simulink model "IFFT64K_2D"  (R2023a)
settings: Solver=VariableStepAuto  StartTime=0.0  StopTime=simtime  RelTol=1e-3
PostLoadFcn:
  | samp_rate = 2e9;
  | fft_sz = 65536;
  | chirp_rate = 200e6 / 1e-3;
  | tone_freq = 20e6;
  | input_bits = 12;
  | align_delay = 3 * fft_sz;
  | buff_init = complex(int32(zeros(256,1)));
  | NSTREAM = 5;
  | simtime = 2.5e-4;
undefined symbols (not defined in the file): S, vsva2197, xcvc1902
libraries: aieBasic x30, aieUtilities x15, hlsBasic x1, dspxfrm3 x1, dspsrcs4 x1, vmcUtilities x1
(part 2 of 2)

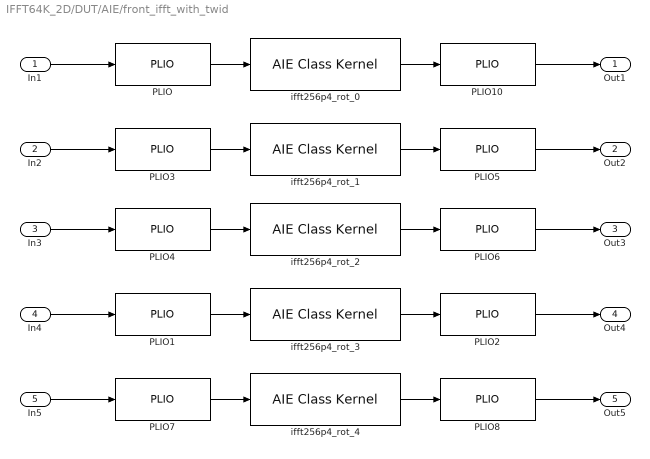
== system IFFT64K_2D/DUT/AIE/front_ifft_with_twid ==
  In1 : Inport
  In2 : Inport  Port=2
  In3 : Inport  Port=3
  In4 : Inport  Port=4
  In5 : Inport  Port=5
  PLIO{,1..8,10} (10 alike) : aieBasic/PLIO  PlioWidth=64  PlioFreqSpec=off  PlioFreq=250  ColLocation=0  channel=0  blockJsonConstraints=[]  deprecateConstraints=0
  ifft256p4_rot_0 : aieBasic/AIE Class Kernel  KernelAllAttrs=|  PortNames={'sig_i'; 'sig_o'}  PortSerializedTypes={'{Q2{R{Tadf::input_buffer{2{t{Scint32}}{t{Tadf::extents{1{t{}260}}}}}}}}'; '{Q2{R{Tadf::output_buffer{2{t{Scint32}}{t{Tadf::extents{1{t{}260}}}}}}}}'}  PortWindowSizes={2.600000000000000000e+02; 2.600000000000000000e+02}  PortWindowMargins={0.000000000000000000e+00; 0.000000000000000000e+00}  PortSynchronicities={'sync', 'sync'}  PortSignalSizes={0.000000000000000000e+00; 0.000000000000000000e+00}  ClassTemplateSpecKind=implicit  ClassTemplateParamNames={'NSTREAM'; 'PHASE'}  ClassTemplateParamKinds={'nontype'; 'nontype'}  ClassTemplateParamTypes={'unsigned int'; 'unsigned int'}  ClassTemplateParamValues={'5', '4'}  ClassCtorParamNames={'tbuff_i'}  ClassCtorParamSerializedTypes={'{R{C{Scint32}256}}'}  ClassCtorParamValues={'[0;0;0;0;0;0;0;0;0;0;0;0;0;0;0;0;0;0;0;0;0;0;0;0;0;0;0;0;0;0;0;0;0;0;0;0;0;0;0;0;0;0;0;0;0;0;0;0;0;0;0;0;0;0;0;0;0;0;0;0;0;0;0;0;0;0;0;0;0;0;0;0;0;0;0;0;0;0;0;0;0;0;0;0;0;0;0;0;0;0;0;0;0;0;0;0;0;0;0;0;0;0;0;0;0;0;0;0;0;0;0;0;0;0;0;0;0;0;0;0;0;0;0;0;0;0;0;0;0;0;0;0;0;0;0;0;0;0;0;0;0;0;0;0;0;0;0;0;0;0;0;0;0;0;0;0;0;0;0;0;0;0;0;0;0;0;0;0;0;0;0;0;0;0;0;0;0;0;0;0;0;0;0;0;0;0;0;0;0;0;0;0;0;0;0;0;0;0;0;0;0;0;0;0;0;0;0;0;0;0;0;0;0;0;0;0;0;0;0;0;0;0;0;0;0;0;0;0;0;0;0;0;0;0;0;0;0;0;0;0;0;0;0;0;0;0;0;0;0;0;0;0;0;0;0;0]'}  ClassIndex=1  ClassCtorIndex=1  ClassTabVisible=on  ClassTemplateParamsVisible=on  ClassCtorDeclVisible=on  ClassCtorParamsVisible=on  FunctionTabVisible=on  FunctionDecl=|  PortAttrs={ 'input', 'sig_i', 'adf::input_buffer< cint32, adf::extents< 260 > > & restrict', '260', '0', 'sync', ''; 'output', 'sig_o', 'adf::output_buffer< cint32, adf::extents< 260 > > & restrict', '260', '', 'sync', '' }  PortAttrsEnables={'off', 'off', 'off', 'off', 'off', 'off', 'off';'off', 'off', 'off', 'off', 'off', 'off', 'off'}  SampleTime=-1  ClassDeclTypeOptions=C[1 1]@t74@template < unsigned int NSTREAM, unsigned int PHASE > class ifft256p4_rot;  ClassDecl=template < unsigned int NSTREAM, unsigned int PHASE > class ifft256p4_rot;  ClassTemplateParams={ 'NSTREAM', 'unsigned int', 'NSTREAM'; 'PHASE', 'unsigned int', '4' }  ClassTemplateParamsEnables={'off', 'off', 'on';'off', 'off', 'on'}  ClassCtorDeclTypeOptions=C[1 1]@t43@ifft256p4_rot(cint32 ( & tbuff_i ) [ 256 ])  ClassCtorDecl=ifft256p4_rot(cint32 ( & tbuff_i ) [ 256 ])  ClassCtorParams={ 'tbuff_i', 'cint32 ( &) [ 256 ]', 'buff_init' }  KernelHeaderFile=aie_src/ifft256p4_rot.h  KernelClassName=ifft256p4_rot  KernelFunction=run  KernelSourceFile=aie_src/ifft256p4_rot.cpp  KernelSearchPaths={}  PreProcOptions={}  blockJsonConstraints=[]
      KernelAllAttrs=|
      | s[12;12;9;9;19;14;21;23;21;23;24;21;15;17;12;24;26;26;26;27;28;9;21;23;23;23;24;25;14;19;19;29]@FunctionNameDeclFileNamePortNamesPortTypesPortSerializedTypesPortDirectionsPortWindowSizeEnablesPortWindowMarginEnablesPortBufferSizeEnablesPortBufferMarginEnablesPortSynchronicityEnablesPortSignalSizeEnablesPortBufferSizesPortBufferMarginsFunctionDeclFunctionTemplateSpecKindFunctionTemplateParamNamesFunctionTemplateParamKindsFunctionTemplateParamTypesFunctionTemplateParamValuesFunctionTemplateParamEnablesClassDeclClassTemplateSpecKindClassTemplateParamNamesClassTemplateParamKindsClassTemplateParamTypesClassTemplateParamValuesClassTemplateParamEnablesClassCtorDeclsClassCtorParamNamesClassCtorParamTypesClassCtorParamSerializedTypes[1 1]@C[32 1]@t3@runt33@../../aie_src/ifft256p4_rot_vmc.hC[2 1]@t5@sig_it5@sig_oC[2 1]@t59@adf::input_buffer< cint32, adf::extents< 260 > > & restrictt60@adf::output_buffer< cint32, adf::extents< 260 > > & restrictC[2 1]@t71@{Q2{R{Tadf::input_buffer{2{t{Scint32}}{t{Tadf::extents{1{t{}260}}}}}}}}t72@{Q2{R{Tadf::output_buffer{2{t{Scint32}}{t{Tadf::extents{1{t{}260}}}}}}}}C[2 1]@t5@inputt6@outputC[2 1]@l1@l1@C[2 1]@l1@l0@C[2 1]@l1@l1@C[2 1]@l0@l0@C[2 1]@l1@l1@C[2 1]@l0@l0@C[2 1]@t3@260t3@260C[2 1]@nnt214@template < unsigned int NSTREAM, unsigned int PHASE > 
      | void ifft256p4_rot::
      | run(adf::input_buffer< cint32, adf::extents< 260 > > & restrict sig_i, adf::output_buffer< cint32, adf::extents< 260 > > & restrict sig_o)t4@nonee[0 1]@e[0 1]@e[0 1]@e[0 1]@e[0 1]@t74@template < unsigned int NSTREAM, unsigned int PHASE > class ifft256p4_rot;t8@implicitC[2 1]@t7@NSTREAMt5@PHASEC[2 1]@t7@nontypet7@nontypeC[2 1]@t12@unsigned intt12@unsigned intC[2 1]@nnC[2 1]@l1@l1@C[1 1]@t43@ifft256p4_rot(cint32 ( & tbuff_i ) [ 256 ])C[1 1]@C[1 1]@t7@tbuff_iC[1 1]@C[1 1]@t19@cint32 ( &) [ 256 ]C[1 1]@C[1 1]@t18@{R{C{Scint32}256}}
      FunctionDecl=|
      | template < unsigned int NSTREAM, unsigned int PHASE > 
      | void ifft256p4_rot::
      | run(adf::input_buffer< cint32, adf::extents< 260 > > & restrict sig_i, adf::output_buffer< cint32, adf::extents< 260 > > & restrict sig_o)
  ifft256p4_rot_1 : aieBasic/AIE Class Kernel  KernelAllAttrs=|  PortNames={'sig_i'; 'sig_o'}  PortSerializedTypes={'{Q2{R{Tadf::input_buffer{2{t{Scint32}}{t{Tadf::extents{1{t{}260}}}}}}}}'; '{Q2{R{Tadf::output_buffer{2{t{Scint32}}{t{Tadf::extents{1{t{}260}}}}}}}}'}  PortWindowSizes={2.600000000000000000e+02; 2.600000000000000000e+02}  PortWindowMargins={0.000000000000000000e+00; 0.000000000000000000e+00}  PortSynchronicities={'sync', 'sync'}  PortSignalSizes={0.000000000000000000e+00; 0.000000000000000000e+00}  ClassTemplateSpecKind=implicit  ClassTemplateParamNames={'NSTREAM'; 'PHASE'}  ClassTemplateParamKinds={'nontype'; 'nontype'}  ClassTemplateParamTypes={'unsigned int'; 'unsigned int'}  ClassTemplateParamValues={'5', '4'}  ClassCtorParamNames={'tbuff_i'}  ClassCtorParamSerializedTypes={'{R{C{Scint32}256}}'}  ClassCtorParamValues={'[0;0;0;0;0;0;0;0;0;0;0;0;0;0;0;0;0;0;0;0;0;0;0;0;0;0;0;0;0;0;0;0;0;0;0;0;0;0;0;0;0;0;0;0;0;0;0;0;0;0;0;0;0;0;0;0;0;0;0;0;0;0;0;0;0;0;0;0;0;0;0;0;0;0;0;0;0;0;0;0;0;0;0;0;0;0;0;0;0;0;0;0;0;0;0;0;0;0;0;0;0;0;0;0;0;0;0;0;0;0;0;0;0;0;0;0;0;0;0;0;0;0;0;0;0;0;0;0;0;0;0;0;0;0;0;0;0;0;0;0;0;0;0;0;0;0;0;0;0;0;0;0;0;0;0;0;0;0;0;0;0;0;0;0;0;0;0;0;0;0;0;0;0;0;0;0;0;0;0;0;0;0;0;0;0;0;0;0;0;0;0;0;0;0;0;0;0;0;0;0;0;0;0;0;0;0;0;0;0;0;0;0;0;0;0;0;0;0;0;0;0;0;0;0;0;0;0;0;0;0;0;0;0;0;0;0;0;0;0;0;0;0;0;0;0;0;0;0;0;0;0;0;0;0;0;0]'}  ClassIndex=1  ClassCtorIndex=1  ClassTabVisible=on  ClassTemplateParamsVisible=on  ClassCtorDeclVisible=on  ClassCtorParamsVisible=on  FunctionTabVisible=on  FunctionDecl=|  PortAttrs={ 'input', 'sig_i', 'adf::input_buffer< cint32, adf::extents< 260 > > & restrict', '260', '0', 'sync', ''; 'output', 'sig_o', 'adf::output_buffer< cint32, adf::extents< 260 > > & restrict', '260', '', 'sync', '' }  PortAttrsEnables={'off', 'off', 'off', 'off', 'off', 'off', 'off';'off', 'off', 'off', 'off', 'off', 'off', 'off'}  SampleTime=-1  ClassDeclTypeOptions=C[1 1]@t74@template < unsigned int NSTREAM, unsigned int PHASE > class ifft256p4_rot;  ClassDecl=template < unsigned int NSTREAM, unsigned int PHASE > class ifft256p4_rot;  ClassTemplateParams={ 'NSTREAM', 'unsigned int', 'NSTREAM'; 'PHASE', 'unsigned int', '4' }  ClassTemplateParamsEnables={'off', 'off', 'on';'off', 'off', 'on'}  ClassCtorDeclTypeOptions=C[1 1]@t43@ifft256p4_rot(cint32 ( & tbuff_i ) [ 256 ])  ClassCtorDecl=ifft256p4_rot(cint32 ( & tbuff_i ) [ 256 ])  ClassCtorParams={ 'tbuff_i', 'cint32 ( &) [ 256 ]', 'buff_init' }  KernelHeaderFile=aie_src/ifft256p4_rot.h  KernelClassName=ifft256p4_rot  KernelFunction=run  KernelSourceFile=aie_src/ifft256p4_rot.cpp  KernelSearchPaths={}  PreProcOptions={}  blockJsonConstraints=[]
      KernelAllAttrs=|
      | s[12;12;9;9;19;14;21;23;21;23;24;21;15;17;12;24;26;26;26;27;28;9;21;23;23;23;24;25;14;19;19;29]@FunctionNameDeclFileNamePortNamesPortTypesPortSerializedTypesPortDirectionsPortWindowSizeEnablesPortWindowMarginEnablesPortBufferSizeEnablesPortBufferMarginEnablesPortSynchronicityEnablesPortSignalSizeEnablesPortBufferSizesPortBufferMarginsFunctionDeclFunctionTemplateSpecKindFunctionTemplateParamNamesFunctionTemplateParamKindsFunctionTemplateParamTypesFunctionTemplateParamValuesFunctionTemplateParamEnablesClassDeclClassTemplateSpecKindClassTemplateParamNamesClassTemplateParamKindsClassTemplateParamTypesClassTemplateParamValuesClassTemplateParamEnablesClassCtorDeclsClassCtorParamNamesClassCtorParamTypesClassCtorParamSerializedTypes[1 1]@C[32 1]@t3@runt33@../../aie_src/ifft256p4_rot_vmc.hC[2 1]@t5@sig_it5@sig_oC[2 1]@t59@adf::input_buffer< cint32, adf::extents< 260 > > & restrictt60@adf::output_buffer< cint32, adf::extents< 260 > > & restrictC[2 1]@t71@{Q2{R{Tadf::input_buffer{2{t{Scint32}}{t{Tadf::extents{1{t{}260}}}}}}}}t72@{Q2{R{Tadf::output_buffer{2{t{Scint32}}{t{Tadf::extents{1{t{}260}}}}}}}}C[2 1]@t5@inputt6@outputC[2 1]@l1@l1@C[2 1]@l1@l0@C[2 1]@l1@l1@C[2 1]@l0@l0@C[2 1]@l1@l1@C[2 1]@l0@l0@C[2 1]@t3@260t3@260C[2 1]@nnt214@template < unsigned int NSTREAM, unsigned int PHASE > 
      | void ifft256p4_rot::
      | run(adf::input_buffer< cint32, adf::extents< 260 > > & restrict sig_i, adf::output_buffer< cint32, adf::extents< 260 > > & restrict sig_o)t4@nonee[0 1]@e[0 1]@e[0 1]@e[0 1]@e[0 1]@t74@template < unsigned int NSTREAM, unsigned int PHASE > class ifft256p4_rot;t8@implicitC[2 1]@t7@NSTREAMt5@PHASEC[2 1]@t7@nontypet7@nontypeC[2 1]@t12@unsigned intt12@unsigned intC[2 1]@nnC[2 1]@l1@l1@C[1 1]@t43@ifft256p4_rot(cint32 ( & tbuff_i ) [ 256 ])C[1 1]@C[1 1]@t7@tbuff_iC[1 1]@C[1 1]@t19@cint32 ( &) [ 256 ]C[1 1]@C[1 1]@t18@{R{C{Scint32}256}}
      FunctionDecl=|
      | template < unsigned int NSTREAM, unsigned int PHASE > 
      | void ifft256p4_rot::
      | run(adf::input_buffer< cint32, adf::extents< 260 > > & restrict sig_i, adf::output_buffer< cint32, adf::extents< 260 > > & restrict sig_o)
  ifft256p4_rot_2 : aieBasic/AIE Class Kernel  KernelAllAttrs=|  PortNames={'sig_i'; 'sig_o'}  PortSerializedTypes={'{Q2{R{Tadf::input_buffer{2{t{Scint32}}{t{Tadf::extents{1{t{}260}}}}}}}}'; '{Q2{R{Tadf::output_buffer{2{t{Scint32}}{t{Tadf::extents{1{t{}260}}}}}}}}'}  PortWindowSizes={2.600000000000000000e+02; 2.600000000000000000e+02}  PortWindowMargins={0.000000000000000000e+00; 0.000000000000000000e+00}  PortSynchronicities={'sync', 'sync'}  PortSignalSizes={0.000000000000000000e+00; 0.000000000000000000e+00}  ClassTemplateSpecKind=implicit  ClassTemplateParamNames={'NSTREAM'; 'PHASE'}  ClassTemplateParamKinds={'nontype'; 'nontype'}  ClassTemplateParamTypes={'unsigned int'; 'unsigned int'}  ClassTemplateParamValues={'5', '4'}  ClassCtorParamNames={'tbuff_i'}  ClassCtorParamSerializedTypes={'{R{C{Scint32}256}}'}  ClassCtorParamValues={'[0;0;0;0;0;0;0;0;0;0;0;0;0;0;0;0;0;0;0;0;0;0;0;0;0;0;0;0;0;0;0;0;0;0;0;0;0;0;0;0;0;0;0;0;0;0;0;0;0;0;0;0;0;0;0;0;0;0;0;0;0;0;0;0;0;0;0;0;0;0;0;0;0;0;0;0;0;0;0;0;0;0;0;0;0;0;0;0;0;0;0;0;0;0;0;0;0;0;0;0;0;0;0;0;0;0;0;0;0;0;0;0;0;0;0;0;0;0;0;0;0;0;0;0;0;0;0;0;0;0;0;0;0;0;0;0;0;0;0;0;0;0;0;0;0;0;0;0;0;0;0;0;0;0;0;0;0;0;0;0;0;0;0;0;0;0;0;0;0;0;0;0;0;0;0;0;0;0;0;0;0;0;0;0;0;0;0;0;0;0;0;0;0;0;0;0;0;0;0;0;0;0;0;0;0;0;0;0;0;0;0;0;0;0;0;0;0;0;0;0;0;0;0;0;0;0;0;0;0;0;0;0;0;0;0;0;0;0;0;0;0;0;0;0;0;0;0;0;0;0;0;0;0;0;0;0]'}  ClassIndex=1  ClassCtorIndex=1  ClassTabVisible=on  ClassTemplateParamsVisible=on  ClassCtorDeclVisible=on  ClassCtorParamsVisible=on  FunctionTabVisible=on  FunctionDecl=|  PortAttrs={ 'input', 'sig_i', 'adf::input_buffer< cint32, adf::extents< 260 > > & restrict', '260', '0', 'sync', ''; 'output', 'sig_o', 'adf::output_buffer< cint32, adf::extents< 260 > > & restrict', '260', '', 'sync', '' }  PortAttrsEnables={'off', 'off', 'off', 'off', 'off', 'off', 'off';'off', 'off', 'off', 'off', 'off', 'off', 'off'}  SampleTime=-1  ClassDeclTypeOptions=C[1 1]@t74@template < unsigned int NSTREAM, unsigned int PHASE > class ifft256p4_rot;  ClassDecl=template < unsigned int NSTREAM, unsigned int PHASE > class ifft256p4_rot;  ClassTemplateParams={ 'NSTREAM', 'unsigned int', 'NSTREAM'; 'PHASE', 'unsigned int', '4' }  ClassTemplateParamsEnables={'off', 'off', 'on';'off', 'off', 'on'}  ClassCtorDeclTypeOptions=C[1 1]@t43@ifft256p4_rot(cint32 ( & tbuff_i ) [ 256 ])  ClassCtorDecl=ifft256p4_rot(cint32 ( & tbuff_i ) [ 256 ])  ClassCtorParams={ 'tbuff_i', 'cint32 ( &) [ 256 ]', 'buff_init' }  KernelHeaderFile=aie_src/ifft256p4_rot.h  KernelClassName=ifft256p4_rot  KernelFunction=run  KernelSourceFile=aie_src/ifft256p4_rot.cpp  KernelSearchPaths={}  PreProcOptions={}  blockJsonConstraints=[]
      KernelAllAttrs=|
      | s[12;12;9;9;19;14;21;23;21;23;24;21;15;17;12;24;26;26;26;27;28;9;21;23;23;23;24;25;14;19;19;29]@FunctionNameDeclFileNamePortNamesPortTypesPortSerializedTypesPortDirectionsPortWindowSizeEnablesPortWindowMarginEnablesPortBufferSizeEnablesPortBufferMarginEnablesPortSynchronicityEnablesPortSignalSizeEnablesPortBufferSizesPortBufferMarginsFunctionDeclFunctionTemplateSpecKindFunctionTemplateParamNamesFunctionTemplateParamKindsFunctionTemplateParamTypesFunctionTemplateParamValuesFunctionTemplateParamEnablesClassDeclClassTemplateSpecKindClassTemplateParamNamesClassTemplateParamKindsClassTemplateParamTypesClassTemplateParamValuesClassTemplateParamEnablesClassCtorDeclsClassCtorParamNamesClassCtorParamTypesClassCtorParamSerializedTypes[1 1]@C[32 1]@t3@runt33@../../aie_src/ifft256p4_rot_vmc.hC[2 1]@t5@sig_it5@sig_oC[2 1]@t59@adf::input_buffer< cint32, adf::extents< 260 > > & restrictt60@adf::output_buffer< cint32, adf::extents< 260 > > & restrictC[2 1]@t71@{Q2{R{Tadf::input_buffer{2{t{Scint32}}{t{Tadf::extents{1{t{}260}}}}}}}}t72@{Q2{R{Tadf::output_buffer{2{t{Scint32}}{t{Tadf::extents{1{t{}260}}}}}}}}C[2 1]@t5@inputt6@outputC[2 1]@l1@l1@C[2 1]@l1@l0@C[2 1]@l1@l1@C[2 1]@l0@l0@C[2 1]@l1@l1@C[2 1]@l0@l0@C[2 1]@t3@260t3@260C[2 1]@nnt214@template < unsigned int NSTREAM, unsigned int PHASE > 
      | void ifft256p4_rot::
      | run(adf::input_buffer< cint32, adf::extents< 260 > > & restrict sig_i, adf::output_buffer< cint32, adf::extents< 260 > > & restrict sig_o)t4@nonee[0 1]@e[0 1]@e[0 1]@e[0 1]@e[0 1]@t74@template < unsigned int NSTREAM, unsigned int PHASE > class ifft256p4_rot;t8@implicitC[2 1]@t7@NSTREAMt5@PHASEC[2 1]@t7@nontypet7@nontypeC[2 1]@t12@unsigned intt12@unsigned intC[2 1]@nnC[2 1]@l1@l1@C[1 1]@t43@ifft256p4_rot(cint32 ( & tbuff_i ) [ 256 ])C[1 1]@C[1 1]@t7@tbuff_iC[1 1]@C[1 1]@t19@cint32 ( &) [ 256 ]C[1 1]@C[1 1]@t18@{R{C{Scint32}256}}
      FunctionDecl=|
      | template < unsigned int NSTREAM, unsigned int PHASE > 
      | void ifft256p4_rot::
      | run(adf::input_buffer< cint32, adf::extents< 260 > > & restrict sig_i, adf::output_buffer< cint32, adf::extents< 260 > > & restrict sig_o)
  ifft256p4_rot_3 : aieBasic/AIE Class Kernel  KernelAllAttrs=|  PortNames={'sig_i'; 'sig_o'}  PortSerializedTypes={'{Q2{R{Tadf::input_buffer{2{t{Scint32}}{t{Tadf::extents{1{t{}260}}}}}}}}'; '{Q2{R{Tadf::output_buffer{2{t{Scint32}}{t{Tadf::extents{1{t{}260}}}}}}}}'}  PortWindowSizes={2.600000000000000000e+02; 2.600000000000000000e+02}  PortWindowMargins={0.000000000000000000e+00; 0.000000000000000000e+00}  PortSynchronicities={'sync', 'sync'}  PortSignalSizes={0.000000000000000000e+00; 0.000000000000000000e+00}  ClassTemplateSpecKind=implicit  ClassTemplateParamNames={'NSTREAM'; 'PHASE'}  ClassTemplateParamKinds={'nontype'; 'nontype'}  ClassTemplateParamTypes={'unsigned int'; 'unsigned int'}  ClassTemplateParamValues={'5', '4'}  ClassCtorParamNames={'tbuff_i'}  ClassCtorParamSerializedTypes={'{R{C{Scint32}256}}'}  ClassCtorParamValues={'[0;0;0;0;0;0;0;0;0;0;0;0;0;0;0;0;0;0;0;0;0;0;0;0;0;0;0;0;0;0;0;0;0;0;0;0;0;0;0;0;0;0;0;0;0;0;0;0;0;0;0;0;0;0;0;0;0;0;0;0;0;0;0;0;0;0;0;0;0;0;0;0;0;0;0;0;0;0;0;0;0;0;0;0;0;0;0;0;0;0;0;0;0;0;0;0;0;0;0;0;0;0;0;0;0;0;0;0;0;0;0;0;0;0;0;0;0;0;0;0;0;0;0;0;0;0;0;0;0;0;0;0;0;0;0;0;0;0;0;0;0;0;0;0;0;0;0;0;0;0;0;0;0;0;0;0;0;0;0;0;0;0;0;0;0;0;0;0;0;0;0;0;0;0;0;0;0;0;0;0;0;0;0;0;0;0;0;0;0;0;0;0;0;0;0;0;0;0;0;0;0;0;0;0;0;0;0;0;0;0;0;0;0;0;0;0;0;0;0;0;0;0;0;0;0;0;0;0;0;0;0;0;0;0;0;0;0;0;0;0;0;0;0;0;0;0;0;0;0;0;0;0;0;0;0;0]'}  ClassIndex=1  ClassCtorIndex=1  ClassTabVisible=on  ClassTemplateParamsVisible=on  ClassCtorDeclVisible=on  ClassCtorParamsVisible=on  FunctionTabVisible=on  FunctionDecl=|  PortAttrs={ 'input', 'sig_i', 'adf::input_buffer< cint32, adf::extents< 260 > > & restrict', '260', '0', 'sync', ''; 'output', 'sig_o', 'adf::output_buffer< cint32, adf::extents< 260 > > & restrict', '260', '', 'sync', '' }  PortAttrsEnables={'off', 'off', 'off', 'off', 'off', 'off', 'off';'off', 'off', 'off', 'off', 'off', 'off', 'off'}  SampleTime=-1  ClassDeclTypeOptions=C[1 1]@t74@template < unsigned int NSTREAM, unsigned int PHASE > class ifft256p4_rot;  ClassDecl=template < unsigned int NSTREAM, unsigned int PHASE > class ifft256p4_rot;  ClassTemplateParams={ 'NSTREAM', 'unsigned int', 'NSTREAM'; 'PHASE', 'unsigned int', '4' }  ClassTemplateParamsEnables={'off', 'off', 'on';'off', 'off', 'on'}  ClassCtorDeclTypeOptions=C[1 1]@t43@ifft256p4_rot(cint32 ( & tbuff_i ) [ 256 ])  ClassCtorDecl=ifft256p4_rot(cint32 ( & tbuff_i ) [ 256 ])  ClassCtorParams={ 'tbuff_i', 'cint32 ( &) [ 256 ]', 'buff_init' }  KernelHeaderFile=aie_src/ifft256p4_rot.h  KernelClassName=ifft256p4_rot  KernelFunction=run  KernelSourceFile=aie_src/ifft256p4_rot.cpp  KernelSearchPaths={}  PreProcOptions={}  blockJsonConstraints=[]
      KernelAllAttrs=|
      | s[12;12;9;9;19;14;21;23;21;23;24;21;15;17;12;24;26;26;26;27;28;9;21;23;23;23;24;25;14;19;19;29]@FunctionNameDeclFileNamePortNamesPortTypesPortSerializedTypesPortDirectionsPortWindowSizeEnablesPortWindowMarginEnablesPortBufferSizeEnablesPortBufferMarginEnablesPortSynchronicityEnablesPortSignalSizeEnablesPortBufferSizesPortBufferMarginsFunctionDeclFunctionTemplateSpecKindFunctionTemplateParamNamesFunctionTemplateParamKindsFunctionTemplateParamTypesFunctionTemplateParamValuesFunctionTemplateParamEnablesClassDeclClassTemplateSpecKindClassTemplateParamNamesClassTemplateParamKindsClassTemplateParamTypesClassTemplateParamValuesClassTemplateParamEnablesClassCtorDeclsClassCtorParamNamesClassCtorParamTypesClassCtorParamSerializedTypes[1 1]@C[32 1]@t3@runt33@../../aie_src/ifft256p4_rot_vmc.hC[2 1]@t5@sig_it5@sig_oC[2 1]@t59@adf::input_buffer< cint32, adf::extents< 260 > > & restrictt60@adf::output_buffer< cint32, adf::extents< 260 > > & restrictC[2 1]@t71@{Q2{R{Tadf::input_buffer{2{t{Scint32}}{t{Tadf::extents{1{t{}260}}}}}}}}t72@{Q2{R{Tadf::output_buffer{2{t{Scint32}}{t{Tadf::extents{1{t{}260}}}}}}}}C[2 1]@t5@inputt6@outputC[2 1]@l1@l1@C[2 1]@l1@l0@C[2 1]@l1@l1@C[2 1]@l0@l0@C[2 1]@l1@l1@C[2 1]@l0@l0@C[2 1]@t3@260t3@260C[2 1]@nnt214@template < unsigned int NSTREAM, unsigned int PHASE > 
      | void ifft256p4_rot::
      | run(adf::input_buffer< cint32, adf::extents< 260 > > & restrict sig_i, adf::output_buffer< cint32, adf::extents< 260 > > & restrict sig_o)t4@nonee[0 1]@e[0 1]@e[0 1]@e[0 1]@e[0 1]@t74@template < unsigned int NSTREAM, unsigned int PHASE > class ifft256p4_rot;t8@implicitC[2 1]@t7@NSTREAMt5@PHASEC[2 1]@t7@nontypet7@nontypeC[2 1]@t12@unsigned intt12@unsigned intC[2 1]@nnC[2 1]@l1@l1@C[1 1]@t43@ifft256p4_rot(cint32 ( & tbuff_i ) [ 256 ])C[1 1]@C[1 1]@t7@tbuff_iC[1 1]@C[1 1]@t19@cint32 ( &) [ 256 ]C[1 1]@C[1 1]@t18@{R{C{Scint32}256}}
      FunctionDecl=|
      | template < unsigned int NSTREAM, unsigned int PHASE > 
      | void ifft256p4_rot::
      | run(adf::input_buffer< cint32, adf::extents< 260 > > & restrict sig_i, adf::output_buffer< cint32, adf::extents< 260 > > & restrict sig_o)
  ifft256p4_rot_4 : aieBasic/AIE Class Kernel  KernelAllAttrs=|  PortNames={'sig_i'; 'sig_o'}  PortSerializedTypes={'{Q2{R{Tadf::input_buffer{2{t{Scint32}}{t{Tadf::extents{1{t{}260}}}}}}}}'; '{Q2{R{Tadf::output_buffer{2{t{Scint32}}{t{Tadf::extents{1{t{}260}}}}}}}}'}  PortWindowSizes={2.600000000000000000e+02; 2.600000000000000000e+02}  PortWindowMargins={0.000000000000000000e+00; 0.000000000000000000e+00}  PortSynchronicities={'sync', 'sync'}  PortSignalSizes={0.000000000000000000e+00; 0.000000000000000000e+00}  ClassTemplateSpecKind=implicit  ClassTemplateParamNames={'NSTREAM'; 'PHASE'}  ClassTemplateParamKinds={'nontype'; 'nontype'}  ClassTemplateParamTypes={'unsigned int'; 'unsigned int'}  ClassTemplateParamValues={'5', '4'}  ClassCtorParamNames={'tbuff_i'}  ClassCtorParamSerializedTypes={'{R{C{Scint32}256}}'}  ClassCtorParamValues={'[0;0;0;0;0;0;0;0;0;0;0;0;0;0;0;0;0;0;0;0;0;0;0;0;0;0;0;0;0;0;0;0;0;0;0;0;0;0;0;0;0;0;0;0;0;0;0;0;0;0;0;0;0;0;0;0;0;0;0;0;0;0;0;0;0;0;0;0;0;0;0;0;0;0;0;0;0;0;0;0;0;0;0;0;0;0;0;0;0;0;0;0;0;0;0;0;0;0;0;0;0;0;0;0;0;0;0;0;0;0;0;0;0;0;0;0;0;0;0;0;0;0;0;0;0;0;0;0;0;0;0;0;0;0;0;0;0;0;0;0;0;0;0;0;0;0;0;0;0;0;0;0;0;0;0;0;0;0;0;0;0;0;0;0;0;0;0;0;0;0;0;0;0;0;0;0;0;0;0;0;0;0;0;0;0;0;0;0;0;0;0;0;0;0;0;0;0;0;0;0;0;0;0;0;0;0;0;0;0;0;0;0;0;0;0;0;0;0;0;0;0;0;0;0;0;0;0;0;0;0;0;0;0;0;0;0;0;0;0;0;0;0;0;0;0;0;0;0;0;0;0;0;0;0;0;0]'}  ClassIndex=1  ClassCtorIndex=1  ClassTabVisible=on  ClassTemplateParamsVisible=on  ClassCtorDeclVisible=on  ClassCtorParamsVisible=on  FunctionTabVisible=on  FunctionDecl=|  PortAttrs={ 'input', 'sig_i', 'adf::input_buffer< cint32, adf::extents< 260 > > & restrict', '260', '0', 'sync', ''; 'output', 'sig_o', 'adf::output_buffer< cint32, adf::extents< 260 > > & restrict', '260', '', 'sync', '' }  PortAttrsEnables={'off', 'off', 'off', 'off', 'off', 'off', 'off';'off', 'off', 'off', 'off', 'off', 'off', 'off'}  SampleTime=-1  ClassDeclTypeOptions=C[1 1]@t74@template < unsigned int NSTREAM, unsigned int PHASE > class ifft256p4_rot;  ClassDecl=template < unsigned int NSTREAM, unsigned int PHASE > class ifft256p4_rot;  ClassTemplateParams={ 'NSTREAM', 'unsigned int', 'NSTREAM'; 'PHASE', 'unsigned int', '4' }  ClassTemplateParamsEnables={'off', 'off', 'on';'off', 'off', 'on'}  ClassCtorDeclTypeOptions=C[1 1]@t43@ifft256p4_rot(cint32 ( & tbuff_i ) [ 256 ])  ClassCtorDecl=ifft256p4_rot(cint32 ( & tbuff_i ) [ 256 ])  ClassCtorParams={ 'tbuff_i', 'cint32 ( &) [ 256 ]', 'buff_init' }  KernelHeaderFile=aie_src/ifft256p4_rot.h  KernelClassName=ifft256p4_rot  KernelFunction=run  KernelSourceFile=aie_src/ifft256p4_rot.cpp  KernelSearchPaths={}  PreProcOptions={}  blockJsonConstraints=[]
      KernelAllAttrs=|
      | s[12;12;9;9;19;14;21;23;21;23;24;21;15;17;12;24;26;26;26;27;28;9;21;23;23;23;24;25;14;19;19;29]@FunctionNameDeclFileNamePortNamesPortTypesPortSerializedTypesPortDirectionsPortWindowSizeEnablesPortWindowMarginEnablesPortBufferSizeEnablesPortBufferMarginEnablesPortSynchronicityEnablesPortSignalSizeEnablesPortBufferSizesPortBufferMarginsFunctionDeclFunctionTemplateSpecKindFunctionTemplateParamNamesFunctionTemplateParamKindsFunctionTemplateParamTypesFunctionTemplateParamValuesFunctionTemplateParamEnablesClassDeclClassTemplateSpecKindClassTemplateParamNamesClassTemplateParamKindsClassTemplateParamTypesClassTemplateParamValuesClassTemplateParamEnablesClassCtorDeclsClassCtorParamNamesClassCtorParamTypesClassCtorParamSerializedTypes[1 1]@C[32 1]@t3@runt33@../../aie_src/ifft256p4_rot_vmc.hC[2 1]@t5@sig_it5@sig_oC[2 1]@t59@adf::input_buffer< cint32, adf::extents< 260 > > & restrictt60@adf::output_buffer< cint32, adf::extents< 260 > > & restrictC[2 1]@t71@{Q2{R{Tadf::input_buffer{2{t{Scint32}}{t{Tadf::extents{1{t{}260}}}}}}}}t72@{Q2{R{Tadf::output_buffer{2{t{Scint32}}{t{Tadf::extents{1{t{}260}}}}}}}}C[2 1]@t5@inputt6@outputC[2 1]@l1@l1@C[2 1]@l1@l0@C[2 1]@l1@l1@C[2 1]@l0@l0@C[2 1]@l1@l1@C[2 1]@l0@l0@C[2 1]@t3@260t3@260C[2 1]@nnt214@template < unsigned int NSTREAM, unsigned int PHASE > 
      | void ifft256p4_rot::
      | run(adf::input_buffer< cint32, adf::extents< 260 > > & restrict sig_i, adf::output_buffer< cint32, adf::extents< 260 > > & restrict sig_o)t4@nonee[0 1]@e[0 1]@e[0 1]@e[0 1]@e[0 1]@t74@template < unsigned int NSTREAM, unsigned int PHASE > class ifft256p4_rot;t8@implicitC[2 1]@t7@NSTREAMt5@PHASEC[2 1]@t7@nontypet7@nontypeC[2 1]@t12@unsigned intt12@unsigned intC[2 1]@nnC[2 1]@l1@l1@C[1 1]@t43@ifft256p4_rot(cint32 ( & tbuff_i ) [ 256 ])C[1 1]@C[1 1]@t7@tbuff_iC[1 1]@C[1 1]@t19@cint32 ( &) [ 256 ]C[1 1]@C[1 1]@t18@{R{C{Scint32}256}}
      FunctionDecl=|
      | template < unsigned int NSTREAM, unsigned int PHASE > 
      | void ifft256p4_rot::
      | run(adf::input_buffer< cint32, adf::extents< 260 > > & restrict sig_i, adf::output_buffer< cint32, adf::extents< 260 > > & restrict sig_o)
  Out1 : Outport
  Out2 : Outport  Port=2
  Out3 : Outport  Port=3
  Out4 : Outport  Port=4
  Out5 : Outport  Port=5
  wires:
  PLIO5/1 -> Out2/1
  ifft256p4_rot_3/1 -> PLIO2/1
  PLIO7/1 -> ifft256p4_rot_4/1
  In2/1 -> PLIO3/1
  PLIO4/1 -> ifft256p4_rot_2/1
  PLIO8/1 -> Out5/1
  PLIO/1 -> ifft256p4_rot_0/1
  PLIO6/1 -> Out3/1
  ifft256p4_rot_1/1 -> PLIO5/1
  PLIO3/1 -> ifft256p4_rot_1/1
  PLIO2/1 -> Out4/1
  In5/1 -> PLIO7/1
  PLIO1/1 -> ifft256p4_rot_3/1
  ifft256p4_rot_0/1 -> PLIO10/1
  In1/1 -> PLIO/1
  ifft256p4_rot_2/1 -> PLIO6/1
  ifft256p4_rot_4/1 -> PLIO8/1
  In3/1 -> PLIO4/1
  PLIO10/1 -> Out1/1
  In4/1 -> PLIO1/1

== matlab function IFFT64K_2D/Enabled Subsystem/MATLAB Function1 ==
  data: u1 input; y output; u2 input; u3 input; u4 input; u5 input
function y = ifft_combine(u1, u2, u3, u4, u5)

persistent idx ymat yp
if isempty(idx)
    idx = 1;
    ymat = complex(zeros(260,260));
    yp = complex(zeros(65536,1));
end

ymat((1:5)+5*(idx-1),:) = [u1.'; u2.'; u3.'; u4.'; u5.'];

if idx == 52
    idx = 1;
    yp = reshape(ymat(1:256,1:256), 65536, 1);
else
    idx = idx + 1;
end

y = double(yp);

== matlab function IFFT64K_2D/MATLAB Function ==
  data: u input; y1 output; y2 output; y3 output; y4 output; y5 output
function [y1, y2, y3, y4, y5] = segment_data(u)

persistent idx um1 um2 um3 um4 um5
if isempty(idx)
    idx = 52;
    um1 = zeros(52,260);
    um2 = zeros(52,260);
    um3 = zeros(52,260);
    um4 = zeros(52,260);
    um5 = zeros(52,260);
end

if idx == 52
    umat = [[reshape(u,256,256); zeros(4,256)] zeros(260,4)];
    um1 = umat(1:5:end,:);
    um2 = umat(2:5:end,:);
    um3 = umat(3:5:end,:);
    um4 = umat(4:5:end,:);
    um5 = umat(5:5:end,:);
    idx = 1;
    y1 = int32(um1(idx,:).');
    y2 = int32(um2(idx,:).');
    y3 = int32(um3(idx,:).');
    y4 = int32(um4(idx,:).');
    y5 = int32(um5(idx,:).');
else
    idx = idx + 1;
    y1 = int32(um1(idx,:).');
    y2 = int32(um2(idx,:).');
    y3 = int32(um3(idx,:).');
    y4 = int32(um4(idx,:).');
    y5 = int32(um5(idx,:).');
end
